simulink model "integrador_trapezoidal_discreto"  (R2023b)
settings: Solver=VariableStepAuto  StartTime=0.0  StopTime=0.001  RelTol=1e-3
values from neighbouring files (symbols this model uses):
  Ts = interp_ts(Ts_ts,t)    [calcular_metricas_operacion.m]
settings Model: Creator=Pc  LastModifiedBy=Pc

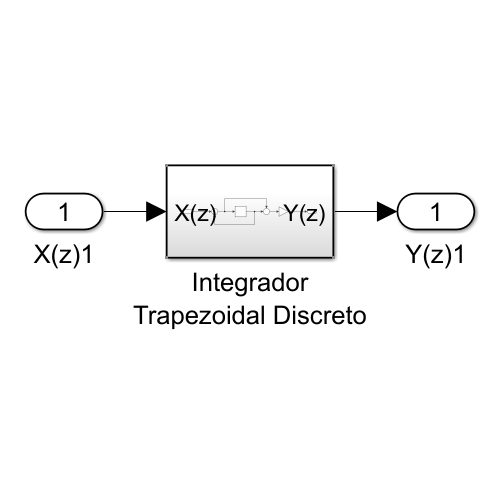
[thumbnail: Simulink's stored preview of the top-level diagram]
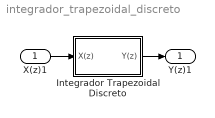
== system integrador_trapezoidal_discreto ==
  X(z)1 : Inport
  Integrador Trapezoidal Discreto : Subsystem
  Y(z)1 : Outport
  wires:
  X(z)1/1 -> Integrador Trapezoidal Discreto/1(X(z))
  Integrador Trapezoidal Discreto/1(Y(z)) -> Y(z)1/1

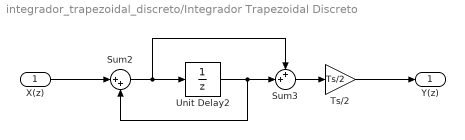
== system integrador_trapezoidal_discreto/Integrador Trapezoidal Discreto ==
  X(z) : Inport
  Sum2 : Sum  Inputs=|++
  Sum3 : Sum  Inputs=++|
  Ts/2 : Gain  Gain=Ts/2
  Unit Delay2 : UnitDelay  SampleTime=-1  HasFrameUpgradeWarning=on
  Y(z) : Outport
  wires:
  Ts/2/1 -> Y(z)/1
  Sum2/1 -> Unit Delay2/1, Sum3/1
  Sum3/1 -> Ts/2/1
  Unit Delay2/1 -> Sum2/2, Sum3/2
  X(z)/1 -> Sum2/1
